simulink model "flightControlSystem"  (R2022b)
settings: Solver=ode3  StartTime=0  StopTime=TFinal  FixedStep=Ts  RelTol=1e-3  EnableMultiTasking=on
undefined symbols (not defined in the file): AltitudeSp, codertarget, Controller, DiscIntNeverNeededParam, Discrete, Estimator, g, gray, init, orient_ref, pos_ref, Sensors, Time, TrackPixlsThrs, Ts, var_acc_angle_N, var_bias_gyr_N, var_gyro_p_N, Vehicle, VelSp
libraries: simulink x39, slpidlib x4, ctrlSharedLib x4, matrix_library x4, sharedtransform x3, parrotlib x1
(part 3 of 3)

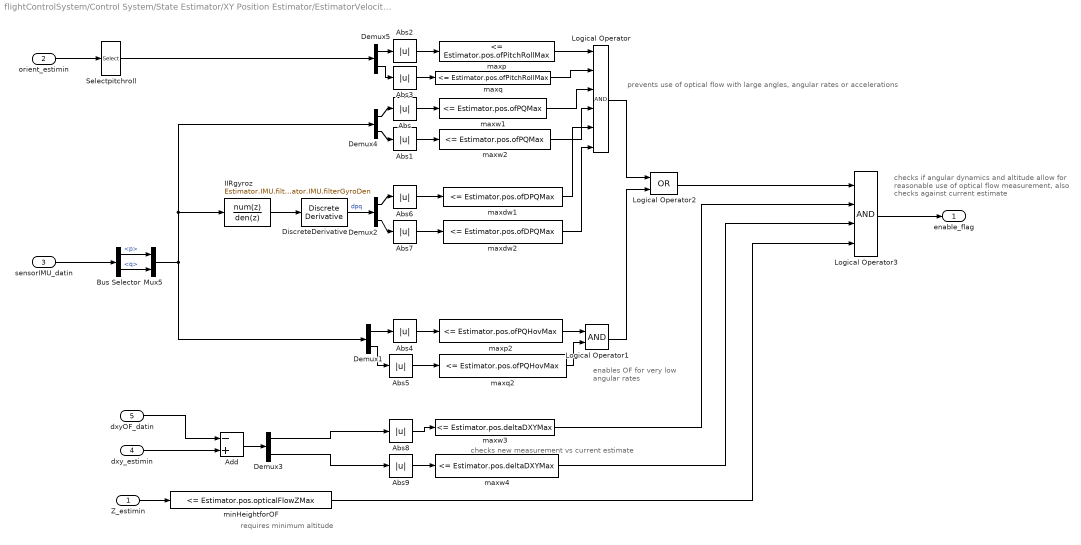
== system flightControlSystem/Control System/State Estimator/XY Position Estimator/EstimatorVelocity/DataHandling ==
  note: prevents use of optical flow with large angles, angular rates or accelerations
  note: enables OF for very
      | low angular rates
  note: checks if angular dynamics and altitude allow for
      | reasonable use of optical flow measurement,
      | also checks against current estimate
  note: checks new measurement vs current estimate
  note: requires minimum altitude
  Z_estimin : Inport
  orient_estimin : Inport  Port=2
  sensorIMU_datin : Inport  Port=3
  dxy_estimin : Inport  Port=4
  dxyOF_datin : Inport  Port=5
  Abs{,1..9} (10 alike) : Abs  SaturateOnIntegerOverflow=off
  Add : Sum  Inputs=-+
  Bus Selector : BusSelector  OutputSignals=p,q
  Demux{1..5} (5 alike) : Demux  Outputs=2
  DiscreteDerivative : simulink/Discrete/Discrete Derivative  gainval=1.0  ICPrevScaledInput=0.0  OutMin=[]  OutMax=[]  OutDataType=fixdt(1, 16)  OutScaling=2^-10  DoSatur=off
  IIRgyroz : DiscreteFilter  Numerator=Estimator.IMU.filterGyroNum  Denominator=Estimator.IMU.filterGyroDen
  Logical Operator : Logic  Inputs=6  AllPortsSameDT=off  OutDataTypeStr=boolean
  Logical Operator1 : Logic  AllPortsSameDT=off  OutDataTypeStr=boolean
  Logical Operator2 : Logic  Operator=OR  AllPortsSameDT=off  OutDataTypeStr=boolean
  Logical Operator3 : Logic  Inputs=4  AllPortsSameDT=off  OutDataTypeStr=boolean
  Mux5 : Mux  Inputs=2
  Selectpitchroll : Selector  InputPortWidth=3  IndexOptions=Index vector (dialog)  Indices=[2 3]  OutputSizes=1
  maxdw1 : simulink/Logic and Bit Operations/Compare To Constant  relop=<=  const=Estimator.pos.ofDPQMax  OutDataTypeStr=boolean
  maxdw2 : simulink/Logic and Bit Operations/Compare To Constant  relop=<=  const=Estimator.pos.ofDPQMax  OutDataTypeStr=boolean
  maxp : simulink/Logic and Bit Operations/Compare To Constant  relop=<=  const=Estimator.pos.ofPitchRollMax  OutDataTypeStr=boolean
  maxp2 : simulink/Logic and Bit Operations/Compare To Constant  relop=<=  const=Estimator.pos.ofPQHovMax  OutDataTypeStr=boolean
  maxq : simulink/Logic and Bit Operations/Compare To Constant  relop=<=  const=Estimator.pos.ofPitchRollMax  OutDataTypeStr=boolean
  maxq2 : simulink/Logic and Bit Operations/Compare To Constant  relop=<=  const=Estimator.pos.ofPQHovMax  OutDataTypeStr=boolean
  maxw1 : simulink/Logic and Bit Operations/Compare To Constant  relop=<=  const=Estimator.pos.ofPQMax  OutDataTypeStr=boolean
  maxw2 : simulink/Logic and Bit Operations/Compare To Constant  relop=<=  const=Estimator.pos.ofPQMax  OutDataTypeStr=boolean
  maxw3 : simulink/Logic and Bit Operations/Compare To Constant  relop=<=  const=Estimator.pos.deltaDXYMax  OutDataTypeStr=boolean
  maxw4 : simulink/Logic and Bit Operations/Compare To Constant  relop=<=  const=Estimator.pos.deltaDXYMax  OutDataTypeStr=boolean
  minHeightforOF : simulink/Logic and Bit Operations/Compare To Constant  relop=<=  const=Estimator.pos.opticalFlowZMax  OutDataTypeStr=boolean
  enable_flag : Outport  VectorParamsAs1DForOutWhenUnconnected=off
  wires:
  minHeightforOF/1 -> Logical Operator3/4
  IIRgyroz/1 -> DiscreteDerivative/1
  Mux5/1 -> Demux1/1, Demux4/1, IIRgyroz/1
  maxw4/1 -> Logical Operator3/3
  maxw3/1 -> Logical Operator3/2
  dxyOF_datin/1 -> Add/1
  Demux3/2 -> Abs9/1
  Demux3/1 -> Abs8/1
  dxy_estimin/1 -> Add/2
  Add/1 -> Demux3/1
  Abs9/1 -> maxw4/1
  Abs8/1 -> maxw3/1
  Logical Operator2/1 -> Logical Operator3/1
  Logical Operator3/1 -> enable_flag/1
  DiscreteDerivative/1 -> Demux2/1  "dpq"
  Demux2/2 -> Abs7/1
  Demux2/1 -> Abs6/1
  Abs7/1 -> maxdw2/1
  Abs6/1 -> maxdw1/1
  Logical Operator1/1 -> Logical Operator2/2
  Demux1/2 -> Abs5/1
  Demux1/1 -> Abs4/1
  Abs5/1 -> maxq2/1
  Abs4/1 -> maxp2/1
  Abs3/1 -> maxq/1
  Abs2/1 -> maxp/1
  Demux4/2 -> Abs1/1
  Demux4/1 -> Abs/1
  Abs1/1 -> maxw2/1
  Abs/1 -> maxw1/1
  Z_estimin/1 -> minHeightforOF/1
  Logical Operator/1 -> Logical Operator2/1
  maxw1/1 -> Logical Operator/3
  Bus Selector/1 -> Mux5/1  "<p>"
  Selectpitchroll/1 -> Demux5/1
  sensorIMU_datin/1 -> Bus Selector/1
  maxq2/1 -> Logical Operator1/2
  Bus Selector/2 -> Mux5/2  "<q>"
  maxp/1 -> Logical Operator/1
  maxw2/1 -> Logical Operator/4
  orient_estimin/1 -> Selectpitchroll/1
  maxdw1/1 -> Logical Operator/5
  maxdw2/1 -> Logical Operator/6
  maxq/1 -> Logical Operator/2
  Demux5/1 -> Abs2/1
  Demux5/2 -> Abs3/1
  maxp2/1 -> Logical Operator1/1

== system flightControlSystem/Control System/State Estimator/XY Position Estimator/EstimatorVelocity/xy velocity w//o angular velocity compensation ==
  note: Optical flow raw readings are converted to velocity in m/s based on the estimated altitude
  optical_flow : Inport
  z_estimate : Inport  Port=2
  " " : Product  Inputs=**
  Compare To Constant : simulink/Logic and Bit Operations/Compare To Constant  relop=<  const=200*4  OutDataTypeStr=boolean
  Counter Free-Running : simulink/Sources/Counter Free-Running  NumBits=32  tsamp=-1
  Gain : Gain  Gain=-1
  Select dxy : Selector  InputPortWidth=3  IndexOptions=Index vector (dialog)  Indices=[1 2]  OutputSizes=1
  Switch : Switch  Criteria=u2 > Threshold  SaturateOnIntegerOverflow=off  InputSameDT=off
  opticalFlowErrorCorrect : Gain  Gain=1.15
  optical_flow_dx_dy : Outport
  wires:
  Select dxy/1 -> optical_flow_dx_dy/1  "optical_flow_dx_dy"
  " "/1 -> opticalFlowErrorCorrect/1
  opticalFlowErrorCorrect/1 -> Switch/3
  Gain/1 -> " "/2
  Switch/1 -> Select dxy/1
  Counter Free-Running/1 -> Compare To Constant/1
  Compare To Constant/1 -> Switch/2
  optical_flow/1 -> " "/1, Switch/1
  z_estimate/1 -> Gain/1

== matlab function flightControlSystem/Control System/Path Planning/LineTrackingAlgorithm/SecondLineTracking/MATLAB Function9 ==
  data: BWimage input; DegAngle output
function DegAngle = FindAngle(BWimage)
edgedBW = edge(BWimage,'canny'); %Canny;
[H, T] = hough(edgedBW); %Hough Transform;
P = houghpeaks(H,2); %peak values;
DegAngle = mean(T(P(:,2))); %found angle value;
end

== matlab function flightControlSystem/Control System/Path Planning/LineTrackingAlgorithm/SecondLineTracking/XYLanding ==
  data: u input; z_final output; x_inc output; C_R input; u_F input; C_B input; y_inc output; Landing_Kill output
function [z_final, x_inc, y_inc, Landing_Kill] = XY_Ctrl(u,C_R,u_F,C_B)
%%%% Tuning parameters
Last_Gain = 0.00035;
Z_gain = 0.0005;
Landing_Final_Size_Circle = 3000;
%%
if C_R == 1 && (u_F(1) == 0 && u_F(2) == 0)
    if C_B <= Landing_Final_Size_Circle
        x_inc = u(1)*Last_Gain;
        y_inc = u(2)*Last_Gain;
    else
        x_inc = 0;
        y_inc = 0;
    end
    Landing_Kill = 1;
    z_final = Z_gain;
else
    Landing_Kill = 0;
    x_inc = 0;
    y_inc = 0;
    z_final = 0;
end

end

== matlab function flightControlSystem/Control System/Path Planning/LineTrackingAlgorithm/SecondLineTracking/XYSlow ==
  data: Trig_End input; x_inc_F output; y_inc_F output; U_prev input; Circle_Detected input; Land_End input
function [x_inc_F, y_inc_F] = XY_Ctrl(Trig_End,U_prev,Circle_Detected,Land_End)
%%%% Tuning parameters
Gain_x_dir = 0.0005;
Gain_y_dir = 0.0005;
%%
    if (Trig_End == 0) && (Circle_Detected == 0) && (Land_End == 0)
        x_inc_F = U_prev(1)*Gain_x_dir;
        y_inc_F = U_prev(2)*Gain_y_dir;
    else
        x_inc_F = 0;
        y_inc_F = 0;
    end
end

== matlab function flightControlSystem/Control System/Path Planning/LineTrackingAlgorithm/SecondLineTracking/XYTrack ==
  data: Trck_ena input; x_inc output; y_inc output; u input
function [x_inc, y_inc] = XY_Ctrl(Trck_ena,u)
%%%% Tuning parameters
Gain_x_dir = 0.001;
Gain_y_dir = 0.001;
%%
    if Trck_ena == 1
        x_inc = u(1)*Gain_x_dir;
        y_inc = u(2)*Gain_y_dir;
    else
        x_inc = 0;
        y_inc = 0;
    end
end

== matlab function flightControlSystem/Image Processing System/LineTrackingAlgorithm/SecondLineTracking/Borderless ==
  data: BW_F input; BW_B_LESS output
function BW_B_LESS = Borderless(BW_F)
% Figures that touch the edge of the image are removed
%%%% Tuning parameters
Border_size = 5;
%%
BW_B_LESS = BW_F;
% Image dimensions
Width = 158;
Height = 118;
% Top edge
BW_F(1:Border_size,1:Width) = BW_F(1:Border_size,1:Width).*-1;
% Bottom edge
BW_F(Height-Border_size+1:Height,1:Width) = BW_F(Height-Border_size+1:Height,1:Width).*-1;
% Left edge
BW_F(Border_size+1:(Height-Border_size),1:Border_size) =...
BW_F(Border_size+1:(Height-Border_size),1:Border_size).*-1;
% Right edge
BW_F(Border_size+1:(Height-Border_size),Width-Border_size+1:Width) =...
BW_F(Border_size+1:(Height-Border_size),Width-Border_size+1:Width).*-1;
% Left - Right Search
for i = Border_size+1:(Height-Border_size)
    for j = Border_size+1:(Width-Border_size)
        if (BW_F(i,j) == 1) && ...
            ((BW_F(i-1,j) == -1) || ...
            (BW_F(i+1,j) == -1) || ...
            (BW_F(i,j-1) == -1) || ...
            (BW_F(i,j+1) == -1) || ...
            (BW_F(i-1,j-1) == -1) || ...
            (BW_F(i-1,j+1) == -1) || ...
            (BW_F(i+1,j-1) == -1) || ...
            (BW_F(i+1,j+1) == -1))
            BW_F(i,j) = -1;
        end
    end
end

% Right - Left Search
for i = (Height-Border_size):-1:Border_size+1 %decreasing
    for j = (Width-Border_size):-1:Border_size+1 %decreasing
        if (BW_F(i,j) == 1) && ...
            ((BW_F(i-1,j) == -1) || ...
            (BW_F(i+1,j) == -1) || ...
            (BW_F(i,j-1) == -1) || ...
            (BW_F(i,j+1) == -1) || ...
            (BW_F(i-1,j-1) == -1) || ...
            (BW_F(i-1,j+1) == -1) || ...
            (BW_F(i+1,j-1) == -1) || ...
            (BW_F(i+1,j+1) == -1))
            BW_F(i,j) = -1;
        end
    end
end

% Down - Top search
for j = (Width-Border_size):-1:Border_size+1 %decreasing
    for i = (Height-Border_size):-1:Border_size+1 %decreasing
        if (BW_F(i,j) == 1) && ...
            ((BW_F(i-1,j) == -1) || ...
            (BW_F(i+1,j) == -1) || ...
            (BW_F(i,j-1) == -1) || ...
            (BW_F(i,j+1) == -1) || ...
            (BW_F(i-1,j-1) == -1) || ...
            (BW_F(i-1,j+1) == -1) || ...
            (BW_F(i+1,j-1) == -1) || ...
            (BW_F(i+1,j+1) == -1))
    
            BW_F(i,j) = -1;
        end
    end
end

% Top - Down search
for j = Border_size+1:(Width-Border_size)
    for i = Border_size+1:(Height-Border_size)
        if (BW_F(i,j) == 1) && ...
            ((BW_F(i-1,j) == -1) || ...
            (BW_F(i+1,j) == -1) || ...
            (BW_F(i,j-1) == -1) || ...
            (BW_F(i,j+1) == -1) || ...
            (BW_F(i-1,j-1) == -1) || ...
            (BW_F(i-1,j+1) == -1) || ...
            (BW_F(i+1,j-1) == -1) || ...
            (BW_F(i+1,j+1) == -1))
    
            BW_F(i,j) = -1;
        end
    end
end

for i = 1:Height
    for j = 1:Width
        if (BW_F(i,j) == -1)
            BW_B_LESS(i,j) = 0;
        end
    end
end

end

== matlab function flightControlSystem/Image Processing System/LineTrackingAlgorithm/SecondLineTracking/CDetFlt ==
  data: BW_B_LESS input; C_DET output; BW_FF output
function [C_DET, BW_FF] = Filter_C_Det(BW_B_LESS)
%%%% Tuning parameters
% The lower is the threshold, the more filtered is the image
Filter_Threshold = 3;
% Pixel threshold to detect circle
C_pixels = 500;
%%
% Image dimensions
Width = 156;
Height = 116;
BW_FF = zeros(Height,Width);
for i = 2:(Height + 1)
    for j = 2:(Width + 1)
        BW_FF(i-1,j-1) = sum(BW_B_LESS(i-1:i+1,j-1:j+1),'all');
        if BW_FF(i-1,j-1) > Filter_Threshold
            BW_FF(i-1,j-1) = 1;
        else
            BW_FF(i-1,j-1) = 0;
        end
    end
end
% Circle detection in the center
    if sum(BW_FF,'all') > C_pixels
        C_DET = 1;
    else
        C_DET = 0;
    end
end

== matlab function flightControlSystem/Image Processing System/LineTrackingAlgorithm/SecondLineTracking/Circle ==
  data: BW_FF input; x_Last output; y_Last output; Sum_end output
function [x_Last, y_Last, Sum_end] = Ctrl_Circle(BW_FF)
%Trying to center the circle to land in the center
% Image dimensions
Width = 156;
Height = 116;
y_inc = sum(BW_FF(:,1:(Width/2)),'all'); %upper half sum
y_dec = sum(BW_FF(:,((Width/2) + 1):Width),'all'); %lower half sum
x_inc = sum(BW_FF(((Height/2)+1):Height,:),'all'); %right half sum
x_dec = sum(BW_FF(1:(Height/2),:),'all'); %left half sum
y_Last = y_dec - y_inc;
x_Last = x_dec - x_inc;
Sum_end = y_inc + y_dec; %whole circle image sum

end

== matlab function flightControlSystem/Image Processing System/LineTrackingAlgorithm/SecondLineTracking/Filter ==
  data: BW input; BW_F output
function BW_F = Filter(BW)
%%%% Tuning Parameters
% The lower is the Threshold, the more filtered is the image
Threshold_Filter = 3;
%%
% Output Image Dimensions
Width = 158;
Height = 118;
BW_F = zeros(Height,Width);
% Filter with a 3x3 box
    for i = 2:(Height + 1)
        for j = 2:(Width + 1)
            BW_F(i-1,j-1) = sum(BW(i-1:i+1,j-1:j+1),'all');
            if BW_F(i-1,j-1) > Threshold_Filter
                BW_F(i-1,j-1) = 1;
            else
                BW_F(i-1,j-1) = 0;
            end
        end
    end
end

== matlab function flightControlSystem/Image Processing System/LineTrackingAlgorithm/SecondLineTracking/MATLAB Function1 ==
  data: BW input; x_incr output; xp input; yp input; y_incr output; Start_End_Flag output
function [x_incr,y_incr,Start_End_Flag] = Ctrl_Radar(BW,xp,yp)
%%%% Tuning parameters
% Radar case size (must be odd dimensions)
% The larger is the size, the more robust is the system
box = 9;
% Detection threshold
Thrs = box*box/2;
% Search Resolution
Red_Srch = 1; %in degrees (1/360)
%%
% Image Dimensions
Width = 158;
Height = 118;
Mag_vec = (Height/2)-((box-1)/2);
Angle_detection = zeros(1,(359+1)/Red_Srch); %it has as many elements as the total degrees (360) divided by the resolution
Angle_detection_centers = zeros(1,(359+1)/Red_Srch);
%Variable for centroid detection
Start_line = 0;
%square and centered matrix
BW2 = BW(:,20:139);
% Circular radar search
for i=0:Red_Srch:359
    y_b_pos = round(Mag_vec*sin(i*pi/180) + Height/2);
    if y_b_pos+((box-1)/2) > Height
        y_b_pos = Height-((box-1)/2);
    elseif (y_b_pos-((box-1)/2) < 1)
        y_b_pos = 1 + ((box-1)/2);
    end

    x_b_pos = round(Height/2 - Mag_vec*cos(i*pi/180));
    if x_b_pos+((box-1)/2) > Height
        x_b_pos = Height-((box-1)/2);
    elseif (x_b_pos-((box-1)/2) < 1)
        x_b_pos = 1 + ((box-1)/2);
    end

    Angle_detection(i+1) = sum(BW2(x_b_pos-((box-1)/2):x_b_pos+((box-1)/2),...
    y_b_pos-((box-1)/2):y_b_pos+((box-1)/2)),'all');
    if Angle_detection(i+1) >= Thrs
        Angle_detection(i+1) = 1;
    else
        Angle_detection(i+1) = 0;
    end
end
% Search for line centers
Angle_detection_Concatenated = [Angle_detection, Angle_detection];
Off_set = 1;
while Angle_detection_Concatenated(Off_set) == 1
    Off_set = Off_set + 1;
end
Angle_detection_Offset = Angle_detection_Concatenated(Off_set:Off_set+359);
White_Line = 0;
Pulse_rise = 0;
Pulse_down = 0;
for i=0:Red_Srch:359
    if (Angle_detection_Offset(i+1) == 1)
    White_Line = White_Line + 1;
    Pulse_rise = 1;
        if (i == 359)
            Pulse_down = 1;
        end
    elseif (Pulse_rise == 1) && (Angle_detection_Offset(i+1) == 0)
        Pulse_down = 1;
        Pulse_rise = 0;
    else
        Pulse_rise = 0;
        Pulse_down = 0;
    end
    if (Pulse_down == 1)
        White_Line = round(White_Line/2);
        Angle_detection_centers(i+1-White_Line) = 1;
        White_Line = 0;
        Pulse_down = 0;
        Pulse_rise = 0;
    end
end
% Detection of all line centers
Points_detected = 6;
x_c_det = 1000*ones(1,Points_detected);
y_c_det = 1000*ones(1,Points_detected);
Actual_pount_found = 1;
for i=0:Red_Srch:359
    if (Angle_detection_centers(i+1) == 1)
        x_c_det(Actual_pount_found) = Mag_vec*cos((i + Off_set)*pi/180);
        y_c_det(Actual_pount_found) = Mag_vec*sin((i + Off_set)*pi/180);
        Actual_pount_found = Actual_pount_found + 1;
    end
    if (Actual_pount_found > Points_detected)
        break;
    end
end
% Distance detection with respect to previous position
Dist_centers_wrt_previous = 1000*ones(1,Points_detected);
for i=1:Points_detected
    Dist_centers_wrt_previous(i) = sqrt((xp - x_c_det(i))^2 +...
    (yp - y_c_det(i))^2);
end
% minimum distance
[Min_dist,Indx_min] = min(Dist_centers_wrt_previous);
if (y_c_det(Indx_min) < 100) && (x_c_det(Indx_min) < 100)
    y_incr = y_c_det(Indx_min);
    x_incr = x_c_det(Indx_min);
else
    y_incr = 0;
    x_incr = 0;
end
if sum(Dist_centers_wrt_previous <= 1000) > 1
    Start_End_Flag = 1;
else
    Start_End_Flag = 0;
end
end

== stateflow chart flightControlSystem/Control System/Path Planning/LineTrackingAlgorithm/LineTracking/Chart ==
  state Hover
    en:
    rot = false;
    du:
    xout = 0;
    yout = 0;
    zout = -0.8;
  state Cruise
    en:
    dx = 0;
    dy = 0;
    land = 0;
    du:
    dx = Vel*cos(YawIn)
    dy = Vel*sin(YawIn)
    xout = xout + dx;
    yout = yout + dy;
    zout = -0.8 ;
  state Rotation
    en:
    rot = true;
    du:
    xout = xout;
    yout = yout;
  (default) -> Hover
  Cruise -> Rotation : [R == true || L == true]
  Hover -> Cruise : [after(4, sec)]{rot = true}
  Rotation -> Cruise : [after(0.5,sec)]{rot = false}
  data: xout output double; yout output double; zout output double; L input; Vel input; YawIn input double; R input; rot output; dy local double; dx local double; land local

== stateflow chart flightControlSystem/Control System/Path Planning/LineTrackingAlgorithm/LineTracking/Chart1 ==
  state Steering
    en:
    OUT==0;
    du:
    if(Left == true)
    OUT = -1;
    elseif(Right == true)
    OUT = 1;
    else
    OUT =0;
    end
  (default) -> Steering
  data: OUT output; Left input; Right input

== matlab function flightControlSystem/Control System/Path Planning/LineTrackingAlgorithm/SecondLineTracking/ZCtrl ==
  data: t_in input; z_sp output; Enab_Go output
function [z_sp, Enab_Go] = Z_Ctrl(t_in)
%%%% Tuning parameters
% SP altitude
Zsp = -0.9;
%%
if (t_in == 1)
    Enab_Go = 1;
else
    Enab_Go = 0;
end

z_sp = Zsp;
end

== matlab function flightControlSystem/Control System/Path Planning/Subsystem1/MATLAB Function9 ==
  data: BWimage input; DegAngle output
function DegAngle = FindAngle(BWimage)
edgedBW = edge(BWimage,'canny'); %Canny;
[H, T] = hough(edgedBW); %Hough Transform;
P = houghpeaks(H,2); %peak values;
DegAngle = mean(T(P(:,2))); %found angle value;
end

== matlab function flightControlSystem/Control System/Path Planning/Subsystem1/XYLanding ==
  data: u input; z_final output; x_inc output; C_R input; u_F input; C_B input; y_inc output; Landing_Kill output
function [z_final, x_inc, y_inc, Landing_Kill] = XY_Ctrl(u,C_R,u_F,C_B)
%%%% Tuning parameters
Last_Gain = 0.00035;
Z_gain = 0.0005;
Landing_Final_Size_Circle = 3000;
%%
if C_R == 1 && (u_F(1) == 0 && u_F(2) == 0)
    if C_B <= Landing_Final_Size_Circle
        x_inc = u(1)*Last_Gain;
        y_inc = u(2)*Last_Gain;
    else
        x_inc = 0;
        y_inc = 0;
    end
    Landing_Kill = 1;
    z_final = Z_gain;
else
    Landing_Kill = 0;
    x_inc = 0;
    y_inc = 0;
    z_final = 0;
end

end

== matlab function flightControlSystem/Image Processing System/detectColorBox ==
  data: RGB input; BW output
function BW  = createMask(RGB)
%createMask  Threshold RGB image using auto-generated code from colorThresholder app.
%  [BW,MASKEDRGBIMAGE] = createMask(RGB) thresholds image RGB using
%  auto-generated code from the colorThresholder app. The colorspace and
%  range for each channel of the colorspace were set within the app. The
%  segmentation mask is returned in BW, and a composite of the mask and
%  original RGB images is returned in maskedRGBImage.

% Auto-generated by colorThresholder app on 28-Apr-2023
%------------------------------------------------------


% Convert RGB image to chosen color space
I = RGB;

% Define thresholds for channel 1 based on histogram settings
channel1Min = 0.000;
channel1Max = 255.000;

% Define thresholds for channel 2 based on histogram settings
channel2Min = 0.000;
channel2Max = 74.000;

% Define thresholds for channel 3 based on histogram settings
channel3Min = 0.000;
channel3Max = 108.000;

% Create mask based on chosen histogram thresholds
sliderBW = (I(:,:,1) >= channel1Min ) & (I(:,:,1) <= channel1Max) & ...
    (I(:,:,2) >= channel2Min ) & (I(:,:,2) <= channel2Max) & ...
    (I(:,:,3) >= channel3Min ) & (I(:,:,3) <= channel3Max);
BW = sliderBW;

% Initialize output masked image based on input image.
maskedRGBImage = RGB;

% Set background pixels where BW is false to zero.
maskedRGBImage(repmat(~BW,[1 1 3])) = 0;

end

== matlab function flightControlSystem/Control System/Path Planning/Subsystem1/XYSlow ==
  data: Trig_End input; x_inc_F output; y_inc_F output; U_prev input; Circle_Detected input; Land_End input
function [x_inc_F, y_inc_F] = XY_Ctrl(Trig_End,U_prev,Circle_Detected,Land_End)
%%%% Tuning parameters
Gain_x_dir = 0.0005;
Gain_y_dir = 0.0005;
%%
    if (Trig_End == 0) && (Circle_Detected == 0) && (Land_End == 0)
        x_inc_F = U_prev(1)*Gain_x_dir;
        y_inc_F = U_prev(2)*Gain_y_dir;
    else
        x_inc_F = 0;
        y_inc_F = 0;
    end
end

== matlab function flightControlSystem/Control System/Path Planning/Subsystem1/XYTrack ==
  data: Trck_ena input; x_inc output; y_inc output; u input
function [x_inc, y_inc] = XY_Ctrl(Trck_ena,u)
%%%% Tuning parameters
Gain_x_dir = 0.001;
Gain_y_dir = 0.001;
%%
    if Trck_ena == 1
        x_inc = u(1)*Gain_x_dir;
        y_inc = u(2)*Gain_y_dir;
    else
        x_inc = 0;
        y_inc = 0;
    end
end

== matlab function flightControlSystem/Control System/Path Planning/Subsystem1/ZCtrl ==
  data: t_in input; z_sp output; Enab_Go output
function [z_sp, Enab_Go] = Z_Ctrl(t_in)
%%%% Tuning parameters
% SP altitude
Zsp = -0.9;
%%
if (t_in == 1)
    Enab_Go = 1;
else
    Enab_Go = 0;
end

z_sp = Zsp;
end

== matlab function flightControlSystem/Control System/Controller/Position Controller/Position error transformation (Earth to Body frame) ==
  data: yaw input; xy_err_earth input; xy_err_body output
function xy_err_body = fcn(yaw,xy_err_earth)

transformation = [cos(yaw), sin(yaw); -sin(yaw),  cos(yaw)];
xy_err_body = transformation * xy_err_earth;


end

== stateflow chart flightControlSystem/Control System/Path Planning/Subsystem1/Subsystem/Chart1 ==
  state Steering
    en:
    OUT==0;
    du:
    if(Left == true)
    OUT = -1;
    elseif(Right == true)
    OUT = 1;
    else
    OUT =0;
    end
  (default) -> Steering
  data: OUT output; Left input; Right input

== matlab function flightControlSystem/Image Processing System/Algorithms/Filter ==
  data: BW input; BW_F output
function BW_F = Filter(BW)
%%%% Tuning Parameters
% The lower is the Threshold, the more filtered is the image
Threshold_Filter = 3;
%%
% Output Image Dimensions
Width = 158;
Height = 118;
BW_F = zeros(Height,Width);
% Filter with a 3x3 box
    for i = 2:(Height + 1)
        for j = 2:(Width + 1)
            BW_F(i-1,j-1) = sum(BW(i-1:i+1,j-1:j+1),'all');
            if BW_F(i-1,j-1) > Threshold_Filter
                BW_F(i-1,j-1) = 1;
            else
                BW_F(i-1,j-1) = 0;
            end
        end
    end
end

== matlab function flightControlSystem/Image Processing System/Algorithms/MATLAB Function1 ==
  data: BW input; x_incr output; xp input; yp input; y_incr output; Start_End_Flag output
function [x_incr,y_incr,Start_End_Flag] = Ctrl_Radar(BW,xp,yp)
%%%% Tuning parameters
% Radar case size (must be odd dimensions)
% The larger is the size, the more robust is the system
box = 9;
% Detection threshold
Thrs = box*box/2;
% Search Resolution
Red_Srch = 1; %in degrees (1/360)
%%
% Image Dimensions
Width = 158;
Height = 118;
Mag_vec = (Height/2)-((box-1)/2);
Angle_detection = zeros(1,(359+1)/Red_Srch); %it has as many elements as the total
degrees (360) divided by the resolution
Angle_detection_centers = zeros(1,(359+1)/Red_Srch);
%Variable for centroid detection
Start_line = 0;
%square and centered matrix
BW2 = BW(:,20:139);
% Circular radar search
for i=0:Red_Srch:359
    y_b_pos = round(Mag_vec*sin(i*pi/180) + Height/2);
    if y_b_pos+((box-1)/2) > Height
        y_b_pos = Height-((box-1)/2);
    elseif (y_b_pos-((box-1)/2) < 1)
        y_b_pos = 1 + ((box-1)/2);
    end

    x_b_pos = round(Height/2 - Mag_vec*cos(i*pi/180));
    if x_b_pos+((box-1)/2) > Height
        x_b_pos = Height-((box-1)/2);
    elseif (x_b_pos-((box-1)/2) < 1)
        x_b_pos = 1 + ((box-1)/2);
    end

    Angle_detection(i+1) = sum(BW2(x_b_pos-((box-1)/2):x_b_pos+((box-1)/2),...
    y_b_pos-((box-1)/2):y_b_pos+((box-1)/2)),'all');
    if Angle_detection(i+1) >= Thrs
        Angle_detection(i+1) = 1;
    else
        Angle_detection(i+1) = 0;
    end
end
% Search for line centers
Angle_detection_Concatenated = [Angle_detection, Angle_detection];
Off_set = 1;
while Angle_detection_Concatenated(Off_set) == 1
    Off_set = Off_set + 1;
end
Angle_detection_Offset = Angle_detection_Concatenated(Off_set:Off_set+359);
White_Line = 0;
Pulse_rise = 0;
Pulse_down = 0;
for i=0:Red_Srch:359
    if (Angle_detection_Offset(i+1) == 1)
    White_Line = White_Line + 1;
    Pulse_rise = 1;
        if (i == 359)
            Pulse_down = 1;
        end
    elseif (Pulse_rise == 1) && (Angle_detection_Offset(i+1) == 0)
        Pulse_down = 1;
        Pulse_rise = 0;
    else
        Pulse_rise = 0;
        Pulse_down = 0;
    end
    if (Pulse_down == 1)
        White_Line = round(White_Line/2);
        Angle_detection_centers(i+1-White_Line) = 1;
        White_Line = 0;
        Pulse_down = 0;
        Pulse_rise = 0;
    end
end
% Detection of all line centers
Points_detected = 6;
x_c_det = 1000*ones(1,Points_detected);
y_c_det = 1000*ones(1,Points_detected);
Actual_pount_found = 1;
for i=0:Red_Srch:359
    if (Angle_detection_centers(i+1) == 1)
        x_c_det(Actual_pount_found) = Mag_vec*cos((i + Off_set)*pi/180);
        y_c_det(Actual_pount_found) = Mag_vec*sin((i + Off_set)*pi/180);
        Actual_pount_found = Actual_pount_found + 1;
    end
    if (Actual_pount_found > Points_detected)
        break;
    end
end
% Distance detection with respect to previous position
Dist_centers_wrt_previous = 1000*ones(1,Points_detected);
for i=1:Points_detected
    Dist_centers_wrt_previous(i) = sqrt((xp - x_c_det(i))^2 +...
    (yp - y_c_det(i))^2);
end
% minimum distance
[Min_dist,Indx_min] = min(Dist_centers_wrt_previous);
if (y_c_det(Indx_min) < 100) && (x_c_det(Indx_min) < 100)
    y_incr = y_c_det(Indx_min);
    x_incr = x_c_det(Indx_min);
else
    y_incr = 0;
    x_incr = 0;
end
if sum(Dist_centers_wrt_previous <= 1000) > 1
    Start_End_Flag = 1;
else
    Start_End_Flag = 0;
end
end

== matlab function flightControlSystem/Image Processing System/Algorithms/Borderless ==
  data: BW_F input; BW_B_LESS output
function BW_B_LESS = Borderless(BW_F)
% Figures that touch the edge of the image are removed
%%%% Tuning parameters
Border_size = 5;
%%
BW_B_LESS = BW_F;
% Image dimensions
Width = 158;
Height = 118;
% Top edge
BW_F(1:Border_size,1:Width) = BW_F(1:Border_size,1:Width).*-1;
% Bottom edge
BW_F(Height-Border_size+1:Height,1:Width) = BW_F(Height-Border_size+1:Height,1:Width).*-
1;
% Left edge
BW_F(Border_size+1:(Height-Border_size),1:Border_size) =...
BW_F(Border_size+1:(Height-Border_size),1:Border_size).*-1;
% Right edge
BW_F(Border_size+1:(Height-Border_size),Width-Border_size+1:Width) =...
BW_F(Border_size+1:(Height-Border_size),Width-Border_size+1:Width).*-1;
% Left - Right Search
for i = Border_size+1:(Height-Border_size)
    for j = Border_size+1:(Width-Border_size)
        if (BW_F(i,j) == 1) && ...
            ((BW_F(i-1,j) == -1) || ...
            (BW_F(i+1,j) == -1) || ...
            (BW_F(i,j-1) == -1) || ...
            (BW_F(i,j+1) == -1) || ...
            (BW_F(i-1,j-1) == -1) || ...
            (BW_F(i-1,j+1) == -1) || ...
            (BW_F(i+1,j-1) == -1) || ...
            (BW_F(i+1,j+1) == -1))
            BW_F(i,j) = -1;
        end
    end
end

% Right - Left Search
for i = (Height-Border_size):-1:Border_size+1 %decreasing
    for j = (Width-Border_size):-1:Border_size+1 %decreasing
        if (BW_F(i,j) == 1) && ...
            ((BW_F(i-1,j) == -1) || ...
            (BW_F(i+1,j) == -1) || ...
            (BW_F(i,j-1) == -1) || ...
            (BW_F(i,j+1) == -1) || ...
            (BW_F(i-1,j-1) == -1) || ...
            (BW_F(i-1,j+1) == -1) || ...
            (BW_F(i+1,j-1) == -1) || ...
            (BW_F(i+1,j+1) == -1))
            BW_F(i,j) = -1;
        end
    end
end

% Down - Top search
for j = (Width-Border_size):-1:Border_size+1 %decreasing
    for i = (Height-Border_size):-1:Border_size+1 %decreasing
        if (BW_F(i,j) == 1) && ...
            ((BW_F(i-1,j) == -1) || ...
            (BW_F(i+1,j) == -1) || ...
            (BW_F(i,j-1) == -1) || ...
            (BW_F(i,j+1) == -1) || ...
            (BW_F(i-1,j-1) == -1) || ...
            (BW_F(i-1,j+1) == -1) || ...
            (BW_F(i+1,j-1) == -1) || ...
            (BW_F(i+1,j+1) == -1))
    
            BW_F(i,j) = -1;
        end
    end
end

% Top - Down search
for j = Border_size+1:(Width-Border_size)
    for i = Border_size+1:(Height-Border_size)
        if (BW_F(i,j) == 1) && ...
            ((BW_F(i-1,j) == -1) || ...
            (BW_F(i+1,j) == -1) || ...
            (BW_F(i,j-1) == -1) || ...
            (BW_F(i,j+1) == -1) || ...
            (BW_F(i-1,j-1) == -1) || ...
            (BW_F(i-1,j+1) == -1) || ...
            (BW_F(i+1,j-1) == -1) || ...
            (BW_F(i+1,j+1) == -1))
    
            BW_F(i,j) = -1;
        end
    end
end

for i = 1:Height
    for j = 1:Width
        if (BW_F(i,j) == -1)
            BW_B_LESS(i,j) = 0;
        end
    end
end

end

== matlab function flightControlSystem/Image Processing System/Algorithms/CDetFlt ==
  data: BW_B_LESS input; C_DET output; BW_FF output
function [C_DET, BW_FF] = Filter_C_Det(BW_B_LESS)
%%%% Tuning parameters
% The lower is the threshold, the more filtered is the image
Filter_Threshold = 3;
% Pixel threshold to detect circle
C_pixels = 500;
%%
% Image dimensions
Width = 156;
Height = 116;
BW_FF = zeros(Height,Width);
for i = 2:(Height + 1)
    for j = 2:(Width + 1)
        BW_FF(i-1,j-1) = sum(BW_B_LESS(i-1:i+1,j-1:j+1),'all');
        if BW_FF(i-1,j-1) > Filter_Threshold
            BW_FF(i-1,j-1) = 1;
        else
            BW_FF(i-1,j-1) = 0;
        end
    end
end
% Circle detection in the center
    if sum(BW_FF,'all') > C_pixels
        C_DET = 1;
    else
        C_DET = 0;
    end
end

== matlab function flightControlSystem/Image Processing System/Algorithms/Circle ==
  data: BW_FF input; x_Last output; y_Last output; Sum_end output
function [x_Last, y_Last, Sum_end] = Ctrl_Circle(BW_FF)
%Trying to center the circle to land in the center
% Image dimensions
Width = 156;
Height = 116;
y_inc = sum(BW_FF(:,1:(Width/2)),'all'); %upper half sum
y_dec = sum(BW_FF(:,((Width/2) + 1):Width),'all'); %lower half sum
x_inc = sum(BW_FF(((Height/2)+1):Height,:),'all'); %right half sum
x_dec = sum(BW_FF(1:(Height/2),:),'all'); %left half sum
y_Last = y_dec - y_inc;
x_Last = x_dec - x_inc;
Sum_end = y_inc + y_dec; %whole circle image sum

end

== stateflow chart flightControlSystem/Control System/Path Planning/Subsystem1/Subsystem/Chart ==
  state Hover
    en:
    rot = false;
    du:
    xout = 0;
    yout = 0;
    zout = -0.8;
  state Cruise
    en:
    dx = 0;
    dy = 0;
    land = 0;
    du:
    dx = (0.00040)*cos(YawIn)
    dy = (0.00040)*sin(YawIn)
    xout = xout + dx;
    yout = yout + dy;
    zout = -0.8 ;
  state Rotation
    en:
    rot = true;
    du:
    xout = xout;
    yout = yout;
  (default) -> Hover
  Cruise -> Rotation : [R == true || L == true]
  Hover -> Cruise : [after(4, sec)]{rot = true}
  Rotation -> Cruise : [after(0.5,sec)]{rot = false}
  data: xout output double; yout output double; zout output double; L input; YawIn input double; R input; rot output; dy local double; dx local double; land local
